simulink model "no3_PI_Controller_22b"  (R2022b)
settings: Solver=FixedStepAuto  StartTime=0.0  StopTime=50  FixedStep=0.2  RelTol=1e-3
libraries: simulink x1
settings Model: Creator=ayeo  LastModifiedBy=ayeo
settings OptimizationCC: ReuseModelBlockBuffer=on
settings RTWCC: GPUComputeCapability=5.0
settings ConfigComp: CovBoundaryAbsTol=1.0e-5

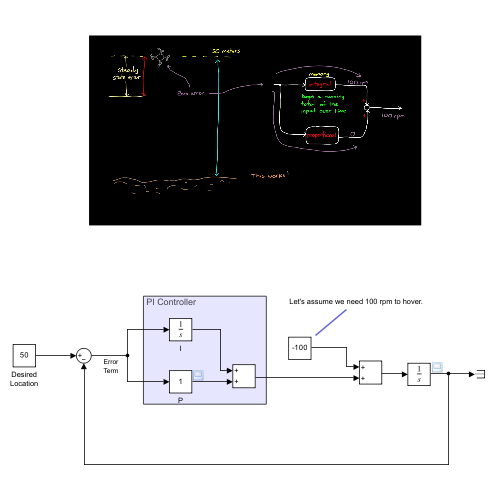
[thumbnail: Simulink's stored preview of the top-level diagram]
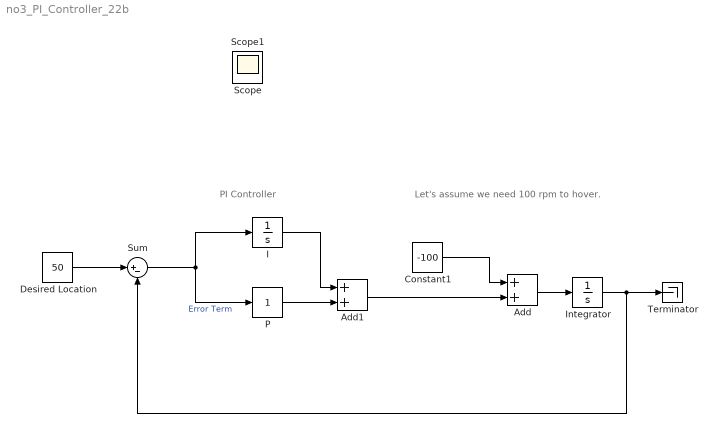
== system no3_PI_Controller_22b ==
  note: Let's assume we need 100 rpm to hover.
  note: PI Controller
  Add : Sum
  Add1 : Sum
  Constant1 : Constant  Value=-100
  Desired Location : Constant  Value=50
  I : Integrator
  Integrator : Integrator
  P : simulink/Math Operations/Slider Gain  gain=1  low=0.1  high=100
  Sum : Sum  Inputs=|+-
  Terminator : Terminator
  Scope : Scope
  Scope1 : Scope
  wires:
  Desired Location/1 -> Sum/1
  Integrator/1 -> Sum/2, Terminator/1
  Add/1 -> Integrator/1
  Constant1/1 -> Add/1
  Add1/1 -> Add/2
  I/1 -> Add1/1
  Sum/1 -> I/1, P/1  "Error Term"
  P/1 -> Add1/2
